simulink model "zad1i2"  (R2023b)
settings: Solver=VariableStepAuto  StartTime=0.0  StopTime=7  RelTol=1e-3
settings Model: Creator=mkmac  LastModifiedBy=Lenovo

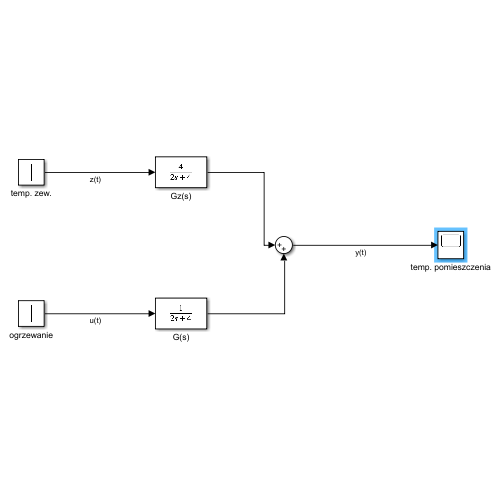
[thumbnail: Simulink's stored preview of the top-level diagram]
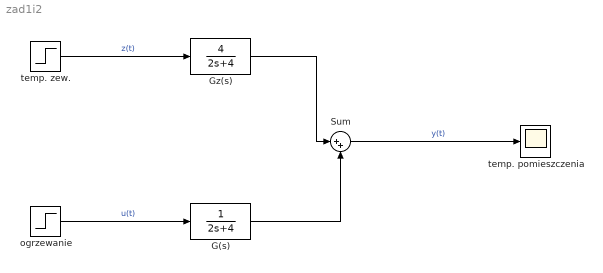
== system zad1i2 ==
  G(s) : TransferFcn  Denominator=[2 4]
  Gz(s) : TransferFcn  Numerator=[4]  Denominator=[2 4]
  Sum : Sum  Inputs=|++
  ogrzewanie : Step  Time=0  After=0  SampleTime=0
  temp. pomieszczenia : Scope
  temp. zew. : Step  Time=2  After=-2  SampleTime=0
  wires:
  temp. zew./1 -> Gz(s)/1  "z(t)"
  ogrzewanie/1 -> G(s)/1  "u(t)"
  G(s)/1 -> Sum/2
  Gz(s)/1 -> Sum/1
  Sum/1 -> temp. pomieszczenia/1  "y(t)"
